simulink model "state_machine_yogurt"  (R2018a)
settings: Solver=FixedStepAuto  StartTime=0.0  StopTime=inf  FixedStep=0.01  RelTol=1e-3
model workspace (MAT data in the model file):
  SL_ROS_VariableLengthArrays_MaxSizes.CommonInfo.ArrayTruncateAction = 'EmitWarning'
  SL_ROS_VariableLengthArrays_MaxSizes.MsgTypeMap = containers.Map
  SL_ROS_VariableLengthArrays_MaxSizes.MsgTypeMap.serialization.keys = {'sensor_msgs/JointState', 'trajectory_msgs/JointTrajectory', 'trajectory_msgs/JointTrajectoryPoint'}
  SL_ROS_VariableLengthArrays_MaxSizes.MsgTypeMap.serialization.values{1}(1).PropertyName = 'Effort'
  SL_ROS_VariableLengthArrays_MaxSizes.MsgTypeMap.serialization.values{1}(1).DataType = 'double'
  SL_ROS_VariableLengthArrays_MaxSizes.MsgTypeMap.serialization.values{1}(1).MaxLength = 7
  SL_ROS_VariableLengthArrays_MaxSizes.MsgTypeMap.serialization.values{1}(2).PropertyName = 'Name'
  SL_ROS_VariableLengthArrays_MaxSizes.MsgTypeMap.serialization.values{1}(2).DataType = 'std_msgs/String'
  SL_ROS_VariableLengthArrays_MaxSizes.MsgTypeMap.serialization.values{1}(2).MaxLength = 16
  SL_ROS_VariableLengthArrays_MaxSizes.MsgTypeMap.serialization.values{1}(3).PropertyName = 'Position'
  SL_ROS_VariableLengthArrays_MaxSizes.MsgTypeMap.serialization.values{1}(3).DataType = 'double'
  SL_ROS_VariableLengthArrays_MaxSizes.MsgTypeMap.serialization.values{1}(3).MaxLength = 7
  SL_ROS_VariableLengthArrays_MaxSizes.MsgTypeMap.serialization.values{1}(4).PropertyName = 'Velocity'
  SL_ROS_VariableLengthArrays_MaxSizes.MsgTypeMap.serialization.values{1}(4).DataType = 'double'
  SL_ROS_VariableLengthArrays_MaxSizes.MsgTypeMap.serialization.values{1}(4).MaxLength = 7
  SL_ROS_VariableLengthArrays_MaxSizes.MsgTypeMap.serialization.values{2}(1).PropertyName = 'JointNames'
  SL_ROS_VariableLengthArrays_MaxSizes.MsgTypeMap.serialization.values{2}(1).DataType = 'std_msgs/String'
  SL_ROS_VariableLengthArrays_MaxSizes.MsgTypeMap.serialization.values{2}(1).MaxLength = 7
  SL_ROS_VariableLengthArrays_MaxSizes.MsgTypeMap.serialization.values{2}(2).PropertyName = 'Points'
  SL_ROS_VariableLengthArrays_MaxSizes.MsgTypeMap.serialization.values{2}(2).DataType = 'trajectory_msgs/JointTrajectoryPoint'
  SL_ROS_VariableLengthArrays_MaxSizes.MsgTypeMap.serialization.values{2}(2).MaxLength = 1
  SL_ROS_VariableLengthArrays_MaxSizes.MsgTypeMap.serialization.values{3}(1).PropertyName = 'Accelerations'
  SL_ROS_VariableLengthArrays_MaxSizes.MsgTypeMap.serialization.values{3}(1).DataType = 'double'
  SL_ROS_VariableLengthArrays_MaxSizes.MsgTypeMap.serialization.values{3}(1).MaxLength = 7
  SL_ROS_VariableLengthArrays_MaxSizes.MsgTypeMap.serialization.values{3}(2).PropertyName = 'Effort'
  SL_ROS_VariableLengthArrays_MaxSizes.MsgTypeMap.serialization.values{3}(2).DataType = 'double'
  SL_ROS_VariableLengthArrays_MaxSizes.MsgTypeMap.serialization.values{3}(2).MaxLength = 7
  SL_ROS_VariableLengthArrays_MaxSizes.MsgTypeMap.serialization.values{3}(3).PropertyName = 'Positions'
  SL_ROS_VariableLengthArrays_MaxSizes.MsgTypeMap.serialization.values{3}(3).DataType = 'double'
  SL_ROS_VariableLengthArrays_MaxSizes.MsgTypeMap.serialization.values{3}(3).MaxLength = 7
  SL_ROS_VariableLengthArrays_MaxSizes.MsgTypeMap.serialization.values{3}(4).PropertyName = 'Velocities'
  SL_ROS_VariableLengthArrays_MaxSizes.MsgTypeMap.serialization.values{3}(4).DataType = 'double'
  SL_ROS_VariableLengthArrays_MaxSizes.MsgTypeMap.serialization.values{3}(4).MaxLength = 7
  SL_ROS_VariableLengthArrays_MaxSizes.MsgTypeMap.serialization.uniformity = 0
  SL_ROS_VariableLengthArrays_MaxSizes.MsgTypeMap.serialization.keyType = 'char'
  SL_ROS_VariableLengthArrays_MaxSizes.MsgTypeMap.serialization.valueType = 'any'
values from neighbouring files (symbols this model uses):
  max_output_len = 4000    [init_yogurt.m]
  pos_threshold = 0.1    [init_yogurt.m]
  t_prova = [2600,2600;1000,1000]    [init_yogurt.m]
undefined symbols (not defined in the file or in its folder): q_0_left, q_0_right
libraries: robotlib x12, realtime_pacer_lib x2
settings Model: Creator=Chiara  LastModifiedBy=kuka

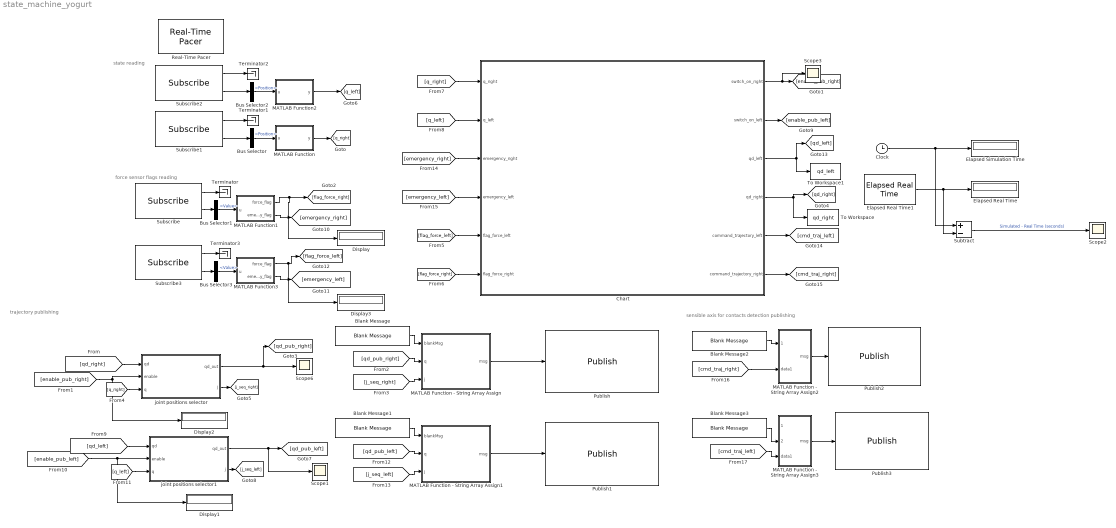
== system state_machine_yogurt ==
  note: sensible axis for contacts detection publishing
  note: trajectory publishing
  note: force sensor flags reading
  note: state reading
  Blank Message : robotlib/Blank Message  SourceLibraryInfo=This block requires Robotics System Toolbox  messageType=trajectory_msgs/JointTrajectory  SampleTime=-1
      settings: SourceProductBaseCode=RO
  Blank Message1 : robotlib/Blank Message  SourceLibraryInfo=This block requires Robotics System Toolbox  messageType=trajectory_msgs/JointTrajectory  SampleTime=-1
      settings: SourceProductBaseCode=RO
  Blank Message2 : robotlib/Blank Message  SourceLibraryInfo=This block requires Robotics System Toolbox  messageType=shared_msgs/CommandTrajectory  SampleTime=-1
      settings: SourceProductBaseCode=RO
  Blank Message3 : robotlib/Blank Message  SourceLibraryInfo=This block requires Robotics System Toolbox  messageType=shared_msgs/CommandTrajectory  SampleTime=-1
      settings: SourceProductBaseCode=RO
  Bus Selector : BusSelector  OutputSignals=Position
  Bus Selector1 : BusSelector  OutputSignals=Value
  Bus Selector2 : BusSelector  OutputSignals=Position
  Bus Selector3 : BusSelector  OutputSignals=Value
  Chart : Stateflow chart  TreatAsAtomicUnit=on
  Clock : Clock
  Display{,1..3} (4 alike) : Display
  Elapsed Real Time : Display
      settings: Decimation=2
  Elapsed Real Time1 : realtime_pacer_lib/Elapsed Real Time
  Elapsed Simulation Time : Display
      settings: Decimation=2
  MATLAB Function : MATLAB Function  TreatAsAtomicUnit=on
  MATLAB Function - String Array Assign : MATLAB Function  TreatAsAtomicUnit=on
  MATLAB Function - String Array Assign1 : MATLAB Function  TreatAsAtomicUnit=on
  MATLAB Function - String Array Assign2 : MATLAB Function  TreatAsAtomicUnit=on
  MATLAB Function - String Array Assign3 : MATLAB Function  TreatAsAtomicUnit=on
  MATLAB Function1 : MATLAB Function  TreatAsAtomicUnit=on
  MATLAB Function2 : MATLAB Function  TreatAsAtomicUnit=on
  MATLAB Function3 : MATLAB Function  TreatAsAtomicUnit=on
  Publish : robotlib/Publish  SourceLibraryInfo=This block requires Robotics System Toolbox  topicSource=Specify your own  topic=/right_arm/command_aux  messageType=trajectory_msgs/JointTrajectory  messageQueueLength=1
      settings: SourceProductBaseCode=RO
  Publish1 : robotlib/Publish  SourceLibraryInfo=This block requires Robotics System Toolbox  topicSource=Specify your own  topic=/left_arm/command_aux  messageType=trajectory_msgs/JointTrajectory  messageQueueLength=1
      settings: SourceProductBaseCode=RO
  Publish2 : robotlib/Publish  SourceLibraryInfo=This block requires Robotics System Toolbox  topicSource=Specify your own  topic=right_arm/command_force_aux  messageType=shared_msgs/CommandTrajectory  messageQueueLength=1
      settings: SourceProductBaseCode=RO
  Publish3 : robotlib/Publish  SourceLibraryInfo=This block requires Robotics System Toolbox  topicSource=Specify your own  topic=left_arm/command_force_aux  messageType=shared_msgs/CommandTrajectory  messageQueueLength=1
      settings: SourceProductBaseCode=RO
  Real-Time Pacer : realtime_pacer_lib/Real-Time Pacer  simTimePerRealTime=1
  Scope{1..3,6} (4 alike) : Scope
  Subscribe : robotlib/Subscribe  SourceLibraryInfo=This block requires Robotics System Toolbox  topicSource=Specify your own  topic=/arms_manager/feedback_force_right  messageType=shared_msgs/FeedbackTrajectory  sampleTime=-1  messageQueueLength=1
      settings: SourceProductBaseCode=RO
  Subscribe1 : robotlib/Subscribe  SourceLibraryInfo=This block requires Robotics System Toolbox  topicSource=Specify your own  topic=/right_arm/joint_states  messageType=sensor_msgs/JointState  sampleTime=-1  messageQueueLength=1
      settings: SourceProductBaseCode=RO
  Subscribe2 : robotlib/Subscribe  SourceLibraryInfo=This block requires Robotics System Toolbox  topicSource=Specify your own  topic=/left_arm/joint_states  messageType=sensor_msgs/JointState  sampleTime=-1  messageQueueLength=1
      settings: SourceProductBaseCode=RO
  Subscribe3 : robotlib/Subscribe  SourceLibraryInfo=This block requires Robotics System Toolbox  topicSource=Specify your own  topic=/arms_manager/feedback_force_left  messageType=shared_msgs/FeedbackTrajectory  sampleTime=-1  messageQueueLength=1
      settings: SourceProductBaseCode=RO
  Subtract : Sum  Inputs=+-
  Terminator{,1..3} (4 alike) : Terminator
  To Workspace : ToWorkspace  VariableName=qd_right  SaveFormat=Timeseries  SampleTime=-1
  To Workspace1 : ToWorkspace  VariableName=qd_left  SaveFormat=Timeseries  SampleTime=-1
  joint positions selector : MATLAB Function  TreatAsAtomicUnit=on
  joint positions selector1 : MATLAB Function  TreatAsAtomicUnit=on
  wires:
  joint positions selector/2(j) -> [j_seq_right]
  joint positions selector/1(qd_out) -> Scope6/1, [qd_pub_right]
  MATLAB Function/1(y) -> [q_right]
  Bus Selector/1 -> MATLAB Function/1(u)  "<Position>"
  [q_right] -> joint positions selector/3(q)
  [enable_pub_right] -> Display2/1, joint positions selector/2(enable)
  Blank Message/1 -> MATLAB Function - String Array Assign/1(blankMsg)
  Subscribe1/2 -> Bus Selector/1
  Bus Selector1/1 -> MATLAB Function1/1(u)  "<Value>"
  [qd_pub_right] -> MATLAB Function - String Array Assign/2(q)
  Subscribe1/1 -> Terminator1/1
  Chart/4(qd_right) -> [qd_right], To Workspace/1
  [qd_right] -> joint positions selector/1(qd)
  Subscribe/2 -> Bus Selector1/1
  MATLAB Function - String Array Assign/1(msg) -> Publish/1
  Subscribe/1 -> Terminator/1
  [j_seq_right] -> MATLAB Function - String Array Assign/3(j)
  [flag_force_left] -> Chart/5(flag_force_left)
  [flag_force_right] -> Chart/6(flag_force_right)
  Chart/1(switch_on_right) -> Scope3/1, [enable_pub_right]
  [q_right] -> Chart/1(q_right)
  MATLAB Function2/1(y) -> [q_left]
  Subscribe2/2 -> Bus Selector2/1
  Bus Selector2/1 -> MATLAB Function2/1(u)  "<Position>"
  Subscribe2/1 -> Terminator2/1
  [q_left] -> Chart/2(q_left)
  [qd_left] -> joint positions selector1/1(qd)
  [enable_pub_left] -> Display1/1, joint positions selector1/2(enable)
  joint positions selector1/1(qd_out) -> [qd_pub_left], Scope1/1
  joint positions selector1/2(j) -> [j_seq_left]
  [q_left] -> joint positions selector1/3(q)
  Chart/2(switch_on_left) -> [enable_pub_left]
  [j_seq_left] -> MATLAB Function - String Array Assign1/3(j)
  [qd_pub_left] -> MATLAB Function - String Array Assign1/2(q)
  MATLAB Function - String Array Assign1/1(msg) -> Publish1/1
  Blank Message1/1 -> MATLAB Function - String Array Assign1/1(blankMsg)
  [emergency_right] -> Chart/3(emergency_right)
  [emergency_left] -> Chart/4(emergency_left)
  MATLAB Function1/2(emergency_flag) -> [emergency_right]
  MATLAB Function3/2(emergency_flag) -> [emergency_left]
  Subscribe3/1 -> Terminator3/1
  Subscribe3/2 -> Bus Selector3/1
  Bus Selector3/1 -> MATLAB Function3/1(u)  "<Value>"
  Chart/3(qd_left) -> [qd_left], To Workspace1/1
  Chart/5(command_trajectory_left) -> [cmd_traj_left]
  Chart/6(command_trajectory_right) -> [cmd_traj_right]
  MATLAB Function - String Array Assign2/1(msg) -> Publish2/1
  Blank Message2/1 -> MATLAB Function - String Array Assign2/1(blankMsg)
  [cmd_traj_right] -> MATLAB Function - String Array Assign2/2(data1)
  [cmd_traj_left] -> MATLAB Function - String Array Assign3/3(data1)
  Blank Message3/1 -> MATLAB Function - String Array Assign3/2(blankMsg)
  MATLAB Function - String Array Assign3/1(msg) -> Publish3/1
  MATLAB Function1/1(force_flag) -> Display/1, [flag_force_right]
  MATLAB Function3/1(force_flag) -> Display3/1, [flag_force_left]
  Clock/1 -> Elapsed Simulation Time/1, Subtract/1
  Elapsed Real Time1/1 -> Elapsed Real Time/1, Subtract/2
  Subtract/1 -> Scope2/1  "Simulated - Real Time (seconds)"

== matlab function state_machine_yogurt/joint positions selector ==
  data: qd input; enable input; qd_out output; j output; q input
function [qd_out, j] = publisher_(qd, enable, q)
%% 
%qd_out = points to be send to the robot
%qd = entire trajectory generated by reverse priority
% enable = equal to 1 once a trajectpry qd has been generated by rev
% priority
%%
% if qd has been generated, this function selects consecutive joint
% positions along the trajectory qd to be send to the robot
persistent count 

if(isempty(count))
    count=0;
end

qd_out = q';

if( enable == 1 )
   count = count + 1;
   if (count > size(qd,2))
       count =  size(qd,2);
   end
   qd_out = qd(:,count);
else
    count = 0;
end
j = count;
end

== matlab function state_machine_yogurt/MATLAB Function ==
  data: u input; y output
function y = fcn(u)
%this function reorder joint position readings 
y = u';
    y(3) = u(7);
    for i = 4 : 7
       y(i) = u(i-1);
    end

== stateflow chart state_machine_yogurt/Chart ==
  settings: updateMethod=DISCRETE  sampleTime=0-01
  state state2
    en:
    q_curr_right = q_right';
    q_curr_left = q_left';
    emergency_flag = 0;
    flag_state = 0;
    %sensible axis for contact or emergency
    command_trajectory_right = [-1 -1 -1 1 -1 -1 ];
    command_trajectory_left = [-1 -1 -1 1 -1 -1 ];
    %flags detecting when the robot has finished its trajetory
    flag_pos_right = 0;
    flag_pos_left = 0;
    coder.extrinsic('spline_traj_left');
    coder.extrinsic('spline_traj_right');
    %flags to state if trajectory has been generated or not yet
    switch_on_right = 0;
    switch_on_left = 0;
    %traj generation
    wp_right2 =[1.4795, 1.1710 - 0.2, 0.9430, -pi/2,0,0];%insert
    wp_left2 =[1.3946, 0.7390+0.2, 0.9069, pi/2, 0,0];%insert
    qd_local_right = spline_traj_right(t_prova(2,1), q_curr_right, wp_right2(1:3)', wp_right2(4:6)',t_prova(2,1));
    qd_local_left = spline_traj_left(t_prova(2,2), q_curr_left, wp_left2(1:3)', wp_left2(4:6)', t_prova(2,2));
    %to have an output that is fixed size(always max_output_len points)
    qd_right = zeros(7,max_output_len);
    qd_left = zeros(7,max_output_len);
    qd_right= [qd_local_right, repmat(qd_local_right(1:7, t_prova(2,1)) ,1, max_output_len-t_prova(2,1))];
    qd_left= [qd_local_left, repmat(qd_local_left(1:7, t_prova(2,2)) ,1, max_output_len-t_prova(2,2))];
    du:
    %sensible axis for contact or emergency
    command_trajectory_right = [2 2 2 1 2 2 ];
    command_trajectory_left = [2 2 2 1 2 2 ];
    switch_on_right = 1;
    switch_on_left = 1;
    err_right=max(abs(angdiff(qd_right(1:7,max_output_len),q_right')));
    err_left = max(abs(angdiff(qd_left(1:7,max_output_len),q_left')));
    if(err_right <= pos_threshold & err_right>0)
    flag_pos_right = 1;
    end
    if(err_left <= pos_threshold & err_left>0)
    flag_pos_left  = 1;
    end
    if((emergency_left || emergency_right)||flag_pos_left||flag_pos_right)
    emergency_flag =1;
    end
    if(flag_force_right && flag_force_left)
    flag_state = 1;
    end
    ex:
    q_curr_right = q_right';
    q_curr_left = q_left';
  state state1
    en:
    flag_state=0;
    emergency_flag=0;
    %sensible axis for contact or emergency
    command_trajectory_right = -1*ones(1,6);
    command_trajectory_left = -1*ones(1,6);
    %flags detecting when the robot has finished its trajetory
    flag_pos_right = 0;
    flag_pos_left = 0;
    coder.extrinsic('spline_traj_left');
    coder.extrinsic('spline_traj_right');
    coder.extrinsic('generate_waypoint');
    %flags to state if trajectory has been generated or not yet
    switch_on_right = 0;
    switch_on_left = 0;
    %traj generation
    %wp_right1 =[  1.5009 ,   1.2710,    1.2214,1.4795 ,   1.1710 ,   0.9430, -pi/2, 0, pi/8];
    %wp_home = generate_waypoint(q_0_right,ones(1,6),zeros(1,6),zeros(1,6));
    wp_right1 =[  1.5009 ,   1.2710,    1.2214,1.4795 ,   1.1710 ,   0.9430, -pi/2,0,0];%insert
    %wp_right1 =[ 0, 0, -pi/2, pi/2, 0, 0];
    %wp_left1 =[0.9939,  1.3420,  0.7951,  1.3946, 1.2420,  0.8769,1.5708 ,  0 , 0, pi/2, pi/20,0];
    wp_left1 =[0.9939,  1.3420,  0.7951,  1.3946, 1.2420,  0.8769,1.5708 ,  pi/2,0,0];%insert
    qd_local_right = spline_traj_right(t_prova(1,1), q_0_right, wp_right1(1:6)', wp_right1(end-2:end)', t_prova(1,1));
    %qd_local_right = spline_traj_right(t_prova(1,1), q_0_right, wp_home(1:3), [0;0;pi/4;0;0;-pi/4], [t_prova(1,1)/2,t_prova(1,1)/2]);
    qd_local_left = spline_traj_left(t_prova(1,2), q_0_left, wp_left1(1:6)', wp_left1(end-2:end)', t_prova(1,2));
    %to have an output that is fixed size(always max_output_len points)
    qd_right = zeros(7,max_output_len);
    qd_left = zeros(7,max_output_len);
    qd_right= [qd_local_right, repmat(qd_local_right(1:7, t_prova(1,1)) ,1, max_output_len-t_prova(1,1))];
    qd_left= [qd_local_left, repmat(qd_local_left(1:7, t_prova(1,2)) ,1, max_output_len-t_prova(1,2))];
    du:
    %sensible axis for contact or emergency
    command_trajectory_right =2* ones(1,6);
    command_trajectory_left = 2*ones(1,6);
    switch_on_right = 1;
    switch_on_left = 1;
    if(emergency_left || emergency_right)
    emergency_flag =1;
    end
    err_right= max(abs(angdiff(qd_right(1:7,max_output_len),q_right')));
    err_left = max(abs(angdiff(qd_left(1:7,max_output_len),q_left')));
    if(err_right <= pos_threshold && err_right~=0)
    flag_pos_right = 1;
    end
    if(err_left <= pos_threshold && err_left~=0)
    flag_pos_left  = 1;
    end
    if(flag_pos_right && flag_pos_left)
    flag_state = 1;
    end
    ex:
    q_curr_right = q_right';
    q_curr_left = q_left';
  state emergency
  state fake_state
  state1 -> state2 [order 1] : [flag_state==1]{switch_on_right=0;switch_on_left = 0; flag_state = 0;}
  (default) -> state1
  state2 -> emergency [order 1] : [emergency_flag==1]{switch_on_left =0; switch_on_right= 0;}
  state2 -> fake_state [order 2] : [flag_state ==1]
  state1 -> emergency [order 2] : [emergency_flag ==1]{switch_on_left =0; switch_on_right = 0;}
  data: pos_threshold parameter; flag_pos local; t_prova parameter; q_0_right parameter; qd_local local; err_left local double; flag_state local; err_right local double; q_right input; q_left input; flag_pos_right local; switch_on_right output; flag_pos_left local; switch_on_left output; qd_left output size=[7 max_output_len]; qd_right output size=[7, max_output_len]; qd_local_right local; qd_local_left local; q_0_left parameter; emergency_right input; emergency_left input; flag_force_left input; flag_force_right input; emergency_flag local; command_trajectory_left output size=[1 6]; command_trajectory_right output size=[1 6]; q_curr_right local; q_curr_left local; wp_right2 local; wp_left2 local; wp_right1 local; wp_left1 local; wp_home local; max_output_len parameter

== matlab function state_machine_yogurt/MATLAB Function1 ==
  data: u input; force_flag output; emergency_flag output
function [force_flag, emergency_flag] = feedback_flags(u)
%this function sets the emergency flag and the "good" contact flag
%according to the F/T sensor reading (u)
switch u
    case 0
        force_flag = 0;
        emergency_flag = 0;
    case 1 
        force_flag = 1;
        emergency_flag = 0;
    otherwise
        force_flag = 0;
        emergency_flag = 1;
end

== matlab function state_machine_yogurt/MATLAB Function2 ==
  data: u input; y output
function y = fcn(u)
%this function reorder joint position readings 
y = u';
    y(3) = u(7);
    for i = 4 : 7
       y(i) = u(i-1);
    end

== matlab function state_machine_yogurt/joint positions selector1 ==
  data: qd input; enable input; qd_out output; j output; q input
function [qd_out, j] = publisher_(qd, enable, q)
%% 
%qd_out = points to be send to the robot
%qd = entire trajectory generated by reverse priority
% enable = equal to 1 once a trajectpry qd has been generated by rev
% priority
%%
% if qd has been generated, this function selects consecutive joint
% positions along the trajectory qd to be send to the robot
persistent count 

if(isempty(count))
    count=0;
end

qd_out = q';

if( enable == 1 )
   count = count + 1;
   if (count > size(qd,2))
       count =  size(qd,2);
   end
   qd_out = qd(:,count);
else
    count = 0;
end
j = count;
end

== matlab function state_machine_yogurt/MATLAB Function - String Array Assign ==
  data: blankMsg input; msg output Bus: SL_Bus_state_machine_yogurt_trajectory_msgs_JointTrajectory; q input; j input
function msg = stringArrayAssign(blankMsg,q,j)
% stringArrayAssign - Assign a string array in a ROS message
%
%  blankMsg (input): A bus for a 'sensor_msgs/JointState' message. This is 
%      used to initialize the output.
%  msg (output): A bus for a 'sensor_msgs/JointState' message message, with 
%      Name field set to a string array.
%
%   Copyright 2015 The MathWorks, Inc.

%#codegen

% Note: The datatype of 'msg' has been explicitly set to the appropriate 
% Simulink bus type ("SL_Bus_robotROSMessageUsageExample_sensor_msgs_JointState"). 
%
% If the model name is changed, the datatype needs to be changed as well:
%   1) Click "Edit Data" in the Editor toolstrip to open "Ports and Data Manager"
%   2) Select "msg". From the "Type" dropdown, select "--- Refresh data types ---"
%   3) Set datatype to "Bus: SL_Bus_<modelname>_sensor_msgs_JointState"

strArrayToAssign = {'right_arm_a1_joint', 'right_arm_a2_joint', 'right_arm_e1_joint', 'right_arm_a3_joint', 'right_arm_a4_joint', 'right_arm_a5_joint', 'right_arm_a6_joint'};
msg = blankMsg;

% Set the number of strings in the string array.
% msg (sensor_msgs/JointState) includes the following fields
%           Name : array of std_msgs/String (string array)
%   Name_SL_Info : struct with fields CurrentLength, ReceivedLength
numStringsInArray = length(strArrayToAssign);
msg.JointNames_SL_Info.CurrentLength = uint32(numStringsInArray);
msg.Points_SL_Info.CurrentLength = uint32(1);
% Set the individual strings in the array
for idx=1:numStringsInArray
    str = strArrayToAssign{idx};
    strLength = length(str);
    msg.JointNames(idx).Data(1:strLength) = uint8(str);
    msg.JointNames(idx).Data_SL_Info.CurrentLength = uint32(strLength);
end
msg.Points(1).Positions(1:length(q)) = q;
msg.Points(1).Positions_SL_Info.CurrentLength = uint32(length(q));
msg.Points(1).TimeFromStart.Sec = 0;
msg.Points(1).TimeFromStart.Nsec = 5000000;

msg.Header.Seq = uint32(j);

== matlab function state_machine_yogurt/MATLAB Function - String Array Assign1 ==
  data: blankMsg input; msg output Bus: SL_Bus_state_machine_yogurt_trajectory_msgs_JointTrajectory; q input; j input
function msg = stringArrayAssign(blankMsg,q,j)
% stringArrayAssign - Assign a string array in a ROS message
%
%  blankMsg (input): A bus for a 'sensor_msgs/JointState' message. This is 
%      used to initialize the output.
%  msg (output): A bus for a 'sensor_msgs/JointState' message message, with 
%      Name field set to a string array.
%
%   Copyleft 2015 The MathWorks, Inc.

%#codegen

% Note: The datatype of 'msg' has been explicitly set to the appropriate 
% Simulink bus type ("SL_Bus_robotROSMessageUsageExample_sensor_msgs_JointState"). 
%
% If the model name is changed, the datatype needs to be changed as well:
%   1) Click "Edit Data" in the Editor toolstrip to open "Ports and Data Manager"
%   2) Select "msg". From the "Type" dropdown, select "--- Refresh data types ---"
%   3) Set datatype to "Bus: SL_Bus_<modelname>_sensor_msgs_JointState"

strArrayToAssign = {'left_arm_a1_joint', 'left_arm_a2_joint', 'left_arm_e1_joint', 'left_arm_a3_joint', 'left_arm_a4_joint', 'left_arm_a5_joint', 'left_arm_a6_joint'};
msg = blankMsg;

% Set the number of strings in the string array.
% msg (sensor_msgs/JointState) includes the following fields
%           Name : array of std_msgs/String (string array)
%   Name_SL_Info : struct with fields CurrentLength, ReceivedLength
numStringsInArray = length(strArrayToAssign);
msg.JointNames_SL_Info.CurrentLength = uint32(numStringsInArray);
msg.Points_SL_Info.CurrentLength = uint32(1);
% Set the individual strings in the array
for idx=1:numStringsInArray
    str = strArrayToAssign{idx};
    strLength = length(str);
    msg.JointNames(idx).Data(1:strLength) = uint8(str);
    msg.JointNames(idx).Data_SL_Info.CurrentLength = uint32(strLength);
end
msg.Points(1).Positions(1:length(q)) = q;
msg.Points(1).Positions_SL_Info.CurrentLength = uint32(length(q));
msg.Points(1).TimeFromStart.Sec = 0;
msg.Points(1).TimeFromStart.Nsec = 5000000;

msg.Header.Seq = uint32(j);

== matlab function state_machine_yogurt/MATLAB Function3 ==
  data: u input; force_flag output; emergency_flag output
function [force_flag, emergency_flag] = feedback_flags(u)
%this function sets the emergency flag and the "good" contact flag
%according to the F/T sensor reading (u)

switch u
    case 0
        force_flag = 0;
        emergency_flag = 0;
    case 1 
        force_flag = 1;
        emergency_flag = 0;
    otherwise
        force_flag = 0;
        emergency_flag = 1;
end

== matlab function state_machine_yogurt/MATLAB Function - String Array Assign2 ==
  data: blankMsg input; msg output Bus: SL_Bus_state_machine_yogurt_shared_msgs_CommandTrajectory; data1 input
function msg = stringArrayAssign(blankMsg,data1)
% stringArrayAssign - Assign a string array in a ROS message
%
%  blankMsg (input): A bus for a 'sensor_msgs/JointState' message. This is 
%      used to initialize the output.
%  msg (output): A bus for a 'sensor_msgs/JointState' message message, with 
%      Name field set to a string array.
%
%   Copyright 2015 The MathWorks, Inc.

%#codegen

% Note: The datatype of 'msg' has been explicitly set to the appropriate 
% Simulink bus type ("SL_Bus_robotROSMessageUsageExample_sensor_msgs_JointState"). 
%
% If the model name is changed, the datatype needs to be changed as well:
%   1) Click "Edit Data" in the Editor toolstrip to open "Ports and Data Manager"
%   2) Select "msg". From the "Type" dropdown, select "--- Refresh data types ---"
%   3) Set datatype to "Bus: SL_Bus_<modelname>_sensor_msgs_JointState"

msg = blankMsg;

% Set the number of strings in the string array.
% msg (sensor_msgs/JointState) includes the following fields
%           Name : array of std_msgs/String (string array)
%   Name_SL_Info : struct with fields CurrentLength, ReceivedLength
% Set the individual strings in the array
msg.FxPos = int8(data1(1));
msg.FxNeg = int8(data1(2));
msg.FyPos = int8(data1(3));
msg.FyNeg = int8(data1(4));
msg.FzPos = int8(data1(5));
msg.FzNeg = int8(data1(6));

== matlab function state_machine_yogurt/MATLAB Function - String Array Assign3 ==
  data: yAssign input; blankMsg input; msg output Bus: SL_Bus_state_machine_yogurt_shared_msgs_CommandTrajectory; data1 input
function msg = stringArra(yAssign,blankMsg,data1)
% stringArrayAssign - Assign a string array in a ROS message
%
%  blankMsg (input): A bus for a 'sensor_msgs/JointState' message. This is 
%      used to initialize the output.
%  msg (output): A bus for a 'sensor_msgs/JointState' message message, with 
%      Name field set to a string array.
%
%   Copyright 2015 The MathWorks, Inc.

%#codegen

% Note: The datatype of 'msg' has been explicitly set to the appropriate 
% Simulink bus type ("SL_Bus_robotROSMessageUsageExample_sensor_msgs_JointState"). 
%
% If the model name is changed, the datatype needs to be changed as well:
%   1) Click "Edit Data" in the Editor toolstrip to open "Ports and Data Manager"
%   2) Select "msg". From the "Type" dropdown, select "--- Refresh data types ---"
%   3) Set datatype to "Bus: SL_Bus_<modelname>_sensor_msgs_JointState"

msg = blankMsg;

% Set the number of strings in the string array.
% msg (sensor_msgs/JointState) includes the following fields
%           Name : array of std_msgs/String (string array)
%   Name_SL_Info : struct with fields CurrentLength, ReceivedLength
% Set the individual strings in the array
msg.FxPos = int8(data1(1));
msg.FxNeg = int8(data1(2));
msg.FyPos = int8(data1(3));
msg.FyNeg = int8(data1(4));
msg.FzPos = int8(data1(5));
msg.FzNeg = int8(data1(6));
